simulink model "test"  (Simulink 6.3)
settings: Solver=ode45  StartTime=0.0  StopTime=10.0  RelTol=1e-3
settings Model: LastModifiedBy=deissenb

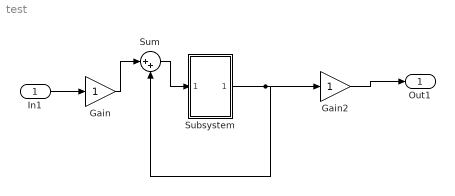
== system test ==
  In1 : Inport
  Gain : Gain
  Gain2 : Gain
  Subsystem : Subsystem
  Sum : Sum  Inputs=|++
  Out1 : Outport
  wires:
  In1/1 -> Gain/1
  Subsystem/1(Out1) -> Gain2/1, Sum/2
  Gain2/1 -> Out1/1
  Gain/1 -> Sum/1
  Sum/1 -> Subsystem/1(In1)

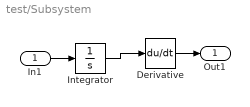
== system test/Subsystem ==
  In1 : Inport
  Derivative : Derivative
  Integrator : Integrator
  Out1 : Outport
  wires:
  Integrator/1 -> Derivative/1
  Derivative/1 -> Out1/1
  In1/1 -> Integrator/1
